simulink model "SimulinkP8_2_Preditor"  (R2018b)
settings: Solver=VariableStepAuto  StartTime=0.0  StopTime=30  RelTol=1e-3
values from neighbouring files (symbols this model uses):
  A = [ 0 1; 0 -3 ]    [Problema8_2.m]
  B = [ 0; 2]    [Problema8_2.m]
  C = [ 1 0 ]    [Problema8_2.m]
  D = 0    [Problema8_2.m]
  h = 0.1    [Problema8_2.m]
  La = [ L Lw ]    [Problema8_2.m]
  Lc = Ganho_DC/( C * inv(eye(2) - phi_cl ) * gama )    [Problema8_2.m]
  p_load = 0.5    [Problema8_2.m]
  t_pert = 20    [Problema8_2.m]
  t_ref = 10    [Problema8_2.m]
  x0 = [ 1; 1]    [Problema8_2.m]
settings Model: Creator=root  LastModifiedBy=root

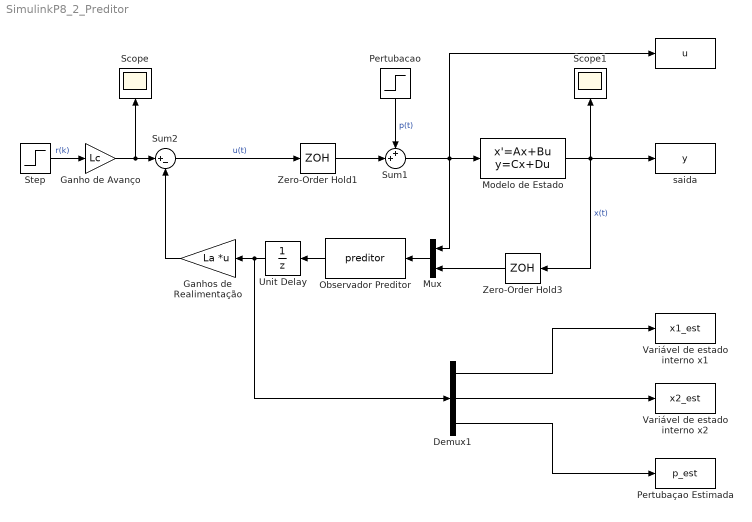
== system SimulinkP8_2_Preditor ==
  " " : ToWorkspace  VariableName=u  SaveFormat=Structure With Time  SampleTime=-1
  " saida" : ToWorkspace  VariableName=y  SaveFormat=Structure With Time  SampleTime=-1
  Demux1 : Demux  Outputs=3
  Ganho de Avanço : Gain  Gain=Lc
  Ganhos de Realimentação : Gain  Gain=La  Multiplication=Matrix(K*u)
  Modelo de Estado : StateSpace  A=A  B=B  C=C  D=D  InitialCondition=x0
  Mux : Mux  Inputs=2
  Observador Preditor : MATLABFcn  MATLABFcn=preditor  OutputDimensions=3
  Pertubacao : Step  Time=t_pert  After=p_load  SampleTime=0
  Pertubaçao Estimada : ToWorkspace  VariableName=p_est  SaveFormat=Structure With Time  SampleTime=-1
  Scope : Scope
  Scope1 : Scope
  Step : Step  Time=t_ref  SampleTime=0
  Sum1 : Sum  Inputs=++|
  Sum2 : Sum  Inputs=|+-
  Unit Delay : UnitDelay  SampleTime=-1
  Variável de estado interno x1 : ToWorkspace  VariableName=x1_est  SaveFormat=Structure With Time  SampleTime=-1
  Variável de estado interno x2 : ToWorkspace  VariableName=x2_est  SaveFormat=Structure With Time  SampleTime=-1
  Zero-Order Hold1 : ZeroOrderHold  SampleTime=h
  Zero-Order Hold3 : ZeroOrderHold  SampleTime=h
  wires:
  Ganhos de Realimentação/1 -> Sum2/2
  Ganho de Avanço/1 -> Sum2/1, Scope/1
  Step/1 -> Ganho de Avanço/1  "r(k)"
  Zero-Order Hold1/1 -> Sum1/2
  Modelo de Estado/1 -> Zero-Order Hold3/1, " saida"/1, Scope1/1  "x(t)"
  Sum1/1 -> Mux/1, " "/1, Modelo de Estado/1
  Pertubacao/1 -> Sum1/1  "p(t)"
  Sum2/1 -> Zero-Order Hold1/1  "u(t)"
  Observador Preditor/1 -> Unit Delay/1
  Unit Delay/1 -> Demux1/1, Ganhos de Realimentação/1
  Mux/1 -> Observador Preditor/1
  Zero-Order Hold3/1 -> Mux/2
  Demux1/1 -> Variável de estado interno x1/1
  Demux1/2 -> Variável de estado interno x2/1
  Demux1/3 -> Pertubaçao Estimada/1
